simulink model "ProblemNo_5"  (R2020b)
settings: Solver=VariableStepAuto  StartTime=0.0  StopTime=10  RelTol=1e-3
settings Model: Creator=Pavan  LastModifiedBy=Pavan

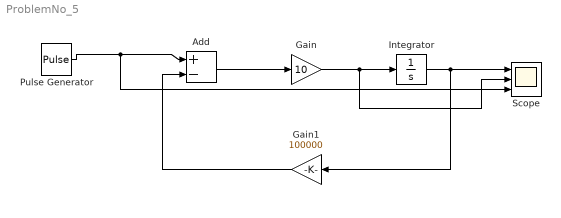
== system ProblemNo_5 ==
  Add : Sum  Inputs=+-
  Gain : Gain  Gain=10
  Gain1 : Gain  Gain=100000
  Integrator : Integrator
  Pulse Generator : DiscretePulseGenerator  PulseType=Time based  Period=7  PulseWidth=2
  Scope : Scope  NumInputPorts=3
  wires:
  Add/1 -> Gain/1
  Integrator/1 -> Gain1/1, Scope/1
  Gain1/1 -> Add/2
  Pulse Generator/1 -> Scope/3, Add/1
  Gain/1 -> Integrator/1, Scope/2
